simulink model "PI_controller_antiwindup2"  (R2019b)
settings: Solver=FixedStepAuto  StartTime=0.0  StopTime=15  FixedStep=0.005  RelTol=1e-3
settings Model: Creator=suvo  LastModifiedBy=suvo

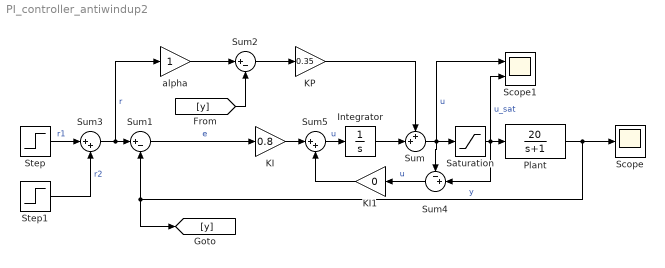
== system PI_controller_antiwindup2 ==
  Integrator : Integrator
  KI : Gain  Gain=0.8
  KI1 : Gain  Gain=0
  KP : Gain  Gain=0.35
  Plant : TransferFcn  Numerator=20  Denominator=[1 1]
  Saturation : Saturate  UpperLimit=0.04  LowerLimit=-0.04
  Scope : Scope
  Scope1 : Scope  NumInputPorts=2
  Step : Step  SampleTime=0
  Step1 : Step  Time=5  After=-1  SampleTime=0
  Sum : Sum  Inputs=++|
  Sum1 : Sum  Inputs=|+-
  Sum2 : Sum  Inputs=|+-
  Sum3 : Sum  Inputs=|++
  Sum4 : Sum  Inputs=-+|
  Sum5 : Sum  Inputs=|++
  alpha : Gain
  wires:
  Plant/1 -> Scope/1, [y], Sum1/2  "y"
  Sum2/1 -> KP/1
  KP/1 -> Sum/1
  Integrator/1 -> Sum/2
  Sum/1 -> Sum4/1, Scope1/1, Saturation/1  "u"
  [y] -> Sum2/2
  alpha/1 -> Sum2/1
  Saturation/1 -> Sum4/2, Plant/1, Scope1/2  "u_sat"
  Step/1 -> Sum3/1  "r1"
  Sum3/1 -> alpha/1, Sum1/1  "r"
  Step1/1 -> Sum3/2  "r2"
  Sum1/1 -> KI/1  "e"
  KI/1 -> Sum5/1
  Sum5/1 -> Integrator/1  "u"
  Sum4/1 -> KI1/1  "u"
  KI1/1 -> Sum5/2
